simulink model "Half_car_model_susp_bump_tyre"  (R2025b)
settings: Solver=VariableStepAuto  StartTime=0.0  StopTime=25  RelTol=1e-3
values from neighbouring files (symbols this model uses):
  A_N = double(vpa(subs(A_0, symbol_vars , numeric_vals), 6))    [half_car_active_suspensions_bump.m]    (also in prova_ordinata.m = vpa(subs(A_0, vars , par), 6))
  B1_N = double(vpa(subs(B1_0, symbol_vars , numeric_vals), 6))    [half_car_active_suspensions_bump.m]    (also in prova_ordinata.m = vpa(subs(B1_0, vars , par), 6))
  B2_N = double(vpa(subs(B2_0, symbol_vars , numeric_vals), 6))    [half_car_active_suspensions_bump.m]    (also in prova_ordinata.m = vpa(subs(B2_0, vars , par), 6))
  C_N = double(vpa(subs(C_0, symbol_vars , numeric_vals), 6))    [half_car_active_suspensions_bump.m]    (also in prova_ordinata.m = vpa(subs(C_0, vars , par), 6))
  CE_N = double(vpa(subs(CE_0, symbol_vars , numeric_vals), 6))    [half_car_active_suspensions_bump.m]    (also in prova_ordinata.m = vpa(subs(CE_0, vars , par), 6))
  D1_N = double(vpa(subs(D1_0, symbol_vars , numeric_vals), 6))    [half_car_active_suspensions_bump.m]    (also in prova_ordinata.m = vpa(subs(D1_0, vars , par), 6))
  D2_N = double(vpa(subs(D2_0, symbol_vars , numeric_vals), 6))    [half_car_active_suspensions_bump.m]    (also in prova_ordinata.m = vpa(subs(D2_0, vars , par), 6))
  DE2_N = double(vpa(subs(DE2_0, symbol_vars , numeric_vals), 6))    [half_car_active_suspensions_bump.m]    (also in prova_ordinata.m = vpa(subs(DE2_0, vars , par), 6))
  Ko = lqr(A_reg', C_N', Q_kalman, R_kalman)'    [half_car_active_suspensions_bump.m]
  Ks = [Ks_c, zeros(2, 4)]    [half_car_active_suspensions_bump.m]
  Ks_obs = -[Ks_lqr_8, zeros(2, 4)]    [half_car_active_suspensions_bump.m]
  par_numeric = [m, kf, kr, betaf, betar, ell0, g, df, dr, J, mwf, mwr, ktf, ktr, hcg]    [half_car_active_suspensions_bump.m]
  rear_bump_time_delay = (df + dr) / vehicle_speed    (= 0.165)    [half_car_active_suspensions_bump.m]
  u0 = [0; 0]    [half_car_active_suspensions_bump.m]    (also in prova_ordinata.m = [0; k * Delta0 * (df - dr)])
  vehicle_speed = 20    [half_car_active_suspensions_bump.m]
  x0 = [  Delta0_num + Delta0_W_num ... (first row only)    [half_car_active_suspensions_bump.m]    (also in prova_ordinata.m = [Delta0)
  x0_lin = [ ... (first row only)    [half_car_active_suspensions_bump.m]
libraries: simulink x1
settings Model: LastModifiedBy=mario

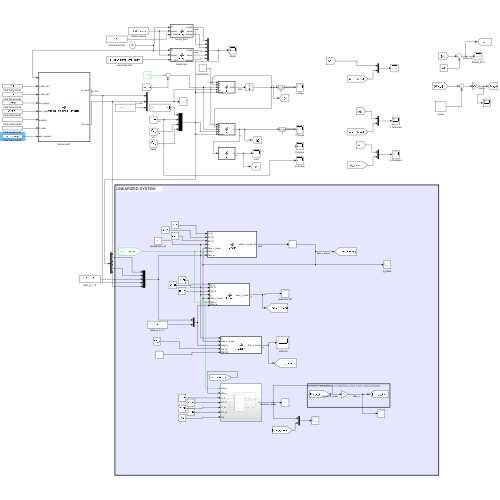
[thumbnail: Simulink's stored preview of the top-level diagram]
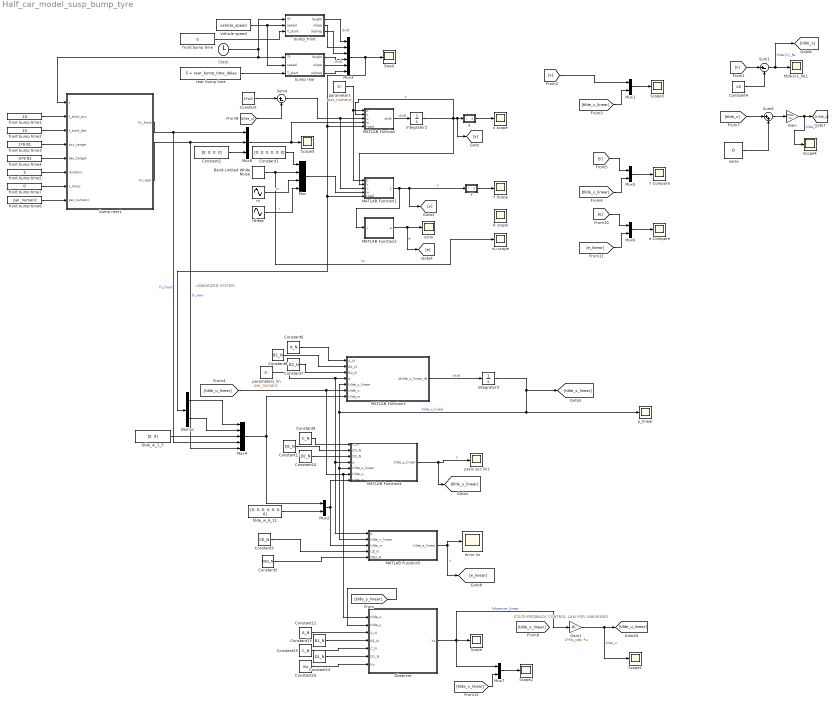
== system Half_car_model_susp_bump_tyre ==
  note: STATE-FEEDBACK CONTROL LAW FOR LINEARISED
  note: LINEARIZED SYSTEM
  " error lin" : Scope
      settings: ActiveDisplayYMinimum=-1  ActiveDisplayYMaximum=1  DataLoggingVariableName=ScopeData8
  Band-Limited White Noise : simulink/Sources/Band-Limited White Noise  Cov="1*[0.00001*1e-2; 0.00001*1e-2;  0.00001*1e-2; 0.00001*1e-2; 0.00001*1e-2]"  Ts=1e-2  seed=[23341; 31826; 11111; 81818; 00001]
  Clock : Clock
  Constant : Constant  Value=1*u0
  Constant1 : Constant  Value=[0; 0; 0; 0; 0; 0]
  Constant10 : Constant  Value=D2_N
  Constant11 : Constant  Value=D1_N
  Constant12 : Constant  Value=A_N
  Constant13 : Constant  Value=B1_N
  Constant14 : Constant  Value=D1_N
  Constant15 : Constant  Value=C_N
  Constant16 : Constant  Value=Ko
  Constant2 : Constant  Value=[0; 0; 0; 0]
  Constant3 : Constant  Value=CE_N
  Constant4 : Constant  Value=x0
  Constant5 : Constant  Value=DE2_N
  Constant6 : Constant  Value=A_N
  Constant7 : Constant  Value=B2_N
  Constant8 : Constant  Value=B1_N
  Constant9 : Constant  Value=C_N
  Demux : Demux  Outputs=6
  Gain : Gain  Gain=0*Ks  Multiplication=Matrix(K*u)
  Gain1 : Gain  Gain=1*Ks_obs  Multiplication=Matrix(K*u)
  Integrator2 : Integrator  InitialCondition=x0
  Integrator3 : Integrator  InitialCondition=x0_lin
  MATLAB Function : MATLAB Function  TreatAsAtomicUnit=on
  MATLAB Function1 : MATLAB Function  TreatAsAtomicUnit=on
  MATLAB Function2 : MATLAB Function  TreatAsAtomicUnit=on
  MATLAB Function3 : MATLAB Function  TreatAsAtomicUnit=on
  MATLAB Function4 : MATLAB Function  TreatAsAtomicUnit=on
  MATLAB Function5 : MATLAB Function  TreatAsAtomicUnit=on
  Mux : Mux
  Mux{1..2,5..7} (5 alike) : Mux  Inputs=2
  Mux3 : Mux  Inputs=6
  Mux4 : Mux  Inputs=5
  Mux8 : Mux  Inputs=3
  Observer : Subsystem
  R scope : Scope
      settings: ActiveDisplayYMinimum=-1  ActiveDisplayYMaximum=1  DataLoggingVariableName=ScopeData5
  Road : Scope
      settings: ActiveDisplayYMinimum=-0.39269908169872414  ActiveDisplayYMaximum=0.39269908169872414
  Scope{,1..5} (6 alike) : Scope
      Scope settings: ActiveDisplayYMinimum=-0.77419611103680575  ActiveDisplayYMaximum=0.44831124007175333  DataLoggingVariableName=ScopeData13
      Scope1 settings: ActiveDisplayYMinimum=-73646.15665947643  ActiveDisplayYMaximum=127134.62422776494  DataLoggingVariableName=ScopeData14
      Scope2 settings: ActiveDisplayYMinimum=-1  ActiveDisplayYMaximum=1  DataLoggingVariableName=ScopeData15
      Scope3 settings: ActiveDisplayYMinimum=-0.11890530130314077  ActiveDisplayYMaximum=0.069183222556784107
      Scope4 settings: ActiveDisplayYMinimum=-1  ActiveDisplayYMaximum=1  DataLoggingVariableName=ScopeData16
      Scope5 settings: ActiveDisplayYMinimum=-18087.1875  ActiveDisplayYMaximum=15634.6875  DataLoggingVariableName=ScopeData17
  Sum1 : Sum  Inputs=|+-
  Sum4 : Sum  Inputs=|+-
  Sum6 : Sum  Inputs=|++
  Vehicle speed : Constant  Value=vehicle_speed  VectorParams1D=off
  X : Subsystem
  Y : Subsystem
  Y Compare : Scope
      settings: ActiveDisplayYMinimum=-9.06978679583773  ActiveDisplayYMaximum=22.15478865739642  DataLoggingVariableName=ScopeData11
  Y Scope : Scope
      settings: ActiveDisplayYMinimum=-1  ActiveDisplayYMaximum=1  DataLoggingVariableName=ScopeData3
  bump rear : MATLAB Function  TreatAsAtomicUnit=on
  bump rear1 : MATLAB Function  TreatAsAtomicUnit=on
  bump_front : MATLAB Function  TreatAsAtomicUnit=on
  e Compare : Scope
      settings: ActiveDisplayYMinimum=-0.3208309292462625  ActiveDisplayYMaximum=0.34771769859425983  DataLoggingVariableName=ScopeData12
  "error " : Scope
      settings: ActiveDisplayYMinimum=-1  ActiveDisplayYMaximum=1  DataLoggingVariableName=ScopeData6
  front bump time : Constant  Value=5  VectorParams1D=off
  front bump time1 : Constant  Value=10  VectorParams1D=off
  front bump time2 : Constant  Value=15  VectorParams1D=off
  front bump time3 : Constant  Value=1*9.81  VectorParams1D=off
  front bump time4 : Constant  Value=-2*9.81  VectorParams1D=off
  front bump time5 : Constant  Value=3  VectorParams1D=off
  front bump time6 : Constant  Value=par_numeric  VectorParams1D=off
  front bump time7 : Constant  Value=0  VectorParams1D=off
  noise : Constant  Value=0
  nu scope : Scope
      settings: DataLoggingVariableName=ScopeData7
  p_linear : Scope
      settings: ActiveDisplayYMinimum=-0.03749851288711617  ActiveDisplayYMaximum=0.066646245320476569  DataLoggingVariableName=ScopeData9
  parameters : Constant  Value=par_numeric  VectorParams1D=off
  parameters_lin : Constant  Value=par_numeric
  rear bump time : Constant  Value=5 + rear_bump_time_delay  VectorParams1D=off
  rtheta : Sin  Amplitude=0  Frequency=0  SampleTime=0
  rz : Sin  Amplitude=0  Frequency=0  SampleTime=0
  tilde_w_1_5 : Constant  Value=[0; 0]
  tilde_w_6_11 : Constant  Value=[0; 0; 0; 0; 0; 0; 0]
  "tilde{x}_NL1" : Scope
      settings: ActiveDisplayYMinimum=-4.93552  ActiveDisplayYMaximum=2.55492  DataLoggingVariableName=ScopeData4
  x scope : Scope
      settings: ActiveDisplayYMinimum=-0.070953530518173463  ActiveDisplayYMaximum=0.13842945478834703  DataLoggingVariableName=ScopeData2
  yaxis acc lin1 : Scope
      settings: ActiveDisplayYMinimum=-1  ActiveDisplayYMaximum=1  DataLoggingVariableName=ScopeData10
  wires:
  Mux3/1 -> MATLAB Function/5(road), Demux/1, MATLAB Function1/5(road), Road/1
  bump_front/1(height) -> Mux3/1  "dxdt"
  Constant/1 -> Sum4/1
  Sum4/1 -> MATLAB Function1/3(u), MATLAB Function/3(u)
  MATLAB Function/1(dxdt) -> Integrator2/1  "dxdt"
  MATLAB Function1/1(y) -> Y/1(i), [y], MATLAB Function2/1(y)  "y"
  rtheta/1 -> Mux/4  "r"
  parameters/1 -> MATLAB Function1/1(p), MATLAB Function/1(p)
  Band-Limited White Noise/1 -> nu scope/1, Mux/2  "nu"
  rz/1 -> Mux/3  "rz"
  Mux/1 -> MATLAB Function1/4(w)
  MATLAB Function2/1(e) -> [e], "error "/1  "e"
  Sum6/1 -> Gain/1
  [tilde_x] -> Sum6/1
  [x] -> Sum1/1
  Constant4/1 -> Sum1/2
  Sum1/1 -> [tilde_x], "tilde{x}_NL1"/1  "tilde{x}_NL"
  noise/1 -> Sum6/2
  [tilde_x_linear] -> Mux1/2
  Gain/1 -> Scope4/1, [tilde_u]  "tilde_u"
  Mux1/1 -> Scope3/1
  [tilde_u] -> Sum4/2
  Integrator2/1 -> [x], X/1(i), MATLAB Function1/2(x), MATLAB Function/2(x)  "x"
  X/1(o) -> x scope/1
  Y/1(o) -> Y Scope/1
  tilde_w_6_11/1 -> Mux2/2
  parameters_lin/1 -> MATLAB Function3/4(p), MATLAB Function5/1(p), MATLAB Function4/4(p)
  [tilde_u_linear] -> MATLAB Function3/6(tilde_u), Observer/1(tilde_u), MATLAB Function4/6(tilde_u)
  Gain1/1 -> Scope1/1, [tilde_u_linear]  "tilde_u"
  MATLAB Function4/1(tilde_y_linear) -> [tilde_y_linear], yaxis acc lin1/1  "y"
  Mux2/1 -> MATLAB Function4/7(tilde_w), MATLAB Function5/3(tilde_w)
  MATLAB Function5/1(tilde_e_linear) -> " error lin"/1, [e_linear]  "y"
  Constant3/1 -> MATLAB Function5/4(CE_N)
  Constant5/1 -> MATLAB Function5/5(DE2_N)
  Constant7/1 -> MATLAB Function3/3(B2_N)
  Constant6/1 -> MATLAB Function3/1(A_N)
  Constant8/1 -> MATLAB Function3/2(B1_N)
  Constant10/1 -> MATLAB Function4/3(D2_N)
  Constant11/1 -> MATLAB Function4/2(D1_N)
  Constant9/1 -> MATLAB Function4/1(C_N)
  Mux4/1 -> MATLAB Function3/7(tilde_w), Mux2/1
  tilde_w_1_5/1 -> Mux4/3
  Demux/2 -> Mux4/1
  Demux/5 -> Mux4/2
  MATLAB Function3/1(dtilde_x_linear_dt) -> Integrator3/1  "dxdt"
  Integrator3/1 -> p_linear/1, MATLAB Function3/5(tilde_x_linear), MATLAB Function5/2(tilde_x_linear), MATLAB Function4/5(tilde_x_linear), [tilde_x_linear]  "tilde_x_linear"
  [y] -> Mux5/1
  Mux5/1 -> Y Compare/1
  [tilde_y_linear] -> Mux5/2
  Mux6/1 -> e Compare/1
  [e] -> Mux6/1
  [e_linear] -> Mux6/2
  [tilde_y_linear] -> Observer/2(tilde_y)
  Observer/1(Yo) -> Mux7/1, Gain1/1, Scope/1  "Yobserver_linear"
  Constant16/1 -> Observer/7(Ko)
  Constant14/1 -> Observer/6(D1_N)
  Constant15/1 -> Observer/5(C_N)
  Constant13/1 -> Observer/4(B1_N)
  Constant12/1 -> Observer/3(A_N)
  Mux7/1 -> Scope2/1
  [x] -> Mux1/1
  bump_front/2(slope) -> Mux3/2
  bump_front/3(alphag) -> Mux3/3
  bump rear/1(height) -> Mux3/4  "dxdt"
  bump rear/2(slope) -> Mux3/5
  bump rear/3(alphag) -> Mux3/6
  Vehicle speed/1 -> bump rear/2(speed), bump_front/2(speed)
  Clock/1 -> bump_front/1(Tf), bump rear/1(Tf), bump rear1/1(t)
  front bump time/1 -> bump_front/3(T_start)
  rear bump time/1 -> bump rear/3(T_start)
  [tilde_x_linear] -> Mux7/2
  front bump time1/1 -> bump rear1/2(t_start_acc)
  front bump time2/1 -> bump rear1/3(t_start_dec)
  front bump time3/1 -> bump rear1/4(acc_target)
  front bump time4/1 -> bump rear1/5(dec_target)
  front bump time5/1 -> bump rear1/6(duration)
  front bump time6/1 -> bump rear1/8(par_numeric)
  bump rear1/1(Fx_front) -> Mux4/4, Mux8/1  "fx_front"
  bump rear1/2(Fx_rear) -> Mux4/5, Mux8/2  "fx_rear"
  Constant1/1 -> Mux/1
  Constant2/1 -> Mux8/3
  Mux8/1 -> Scope5/1, MATLAB Function/4(w)
  front bump time7/1 -> bump rear1/7(t_ramp)

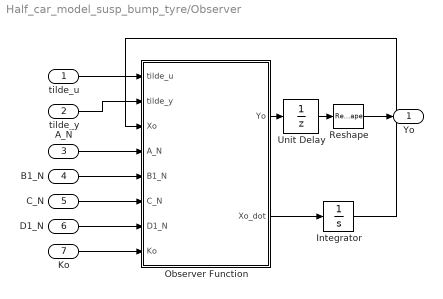
== system Half_car_model_susp_bump_tyre/Observer ==
  tilde_u : Inport
  tilde_y : Inport  Port=2
  A_N : Inport  Port=3
  B1_N : Inport  Port=4
  C_N : Inport  Port=5
  D1_N : Inport  Port=6
  Ko : Inport  Port=7
  Integrator : Integrator  InitialCondition=x0_lin
  Observer Function : MATLAB Function  TreatAsAtomicUnit=on
  Reshape : Reshape  OutputDimensionality=Customize  OutputDimensions=[12]
  Unit Delay : UnitDelay  SampleTime=0.01  HasFrameUpgradeWarning=on
  Yo : Outport
  wires:
  Observer Function/2(Xo_dot) -> Integrator/1
  Integrator/1 -> Observer Function/3(Xo)
  tilde_u/1 -> Observer Function/1(tilde_u)
  tilde_y/1 -> Observer Function/2(tilde_y)
  A_N/1 -> Observer Function/4(A_N)
  B1_N/1 -> Observer Function/5(B1_N)
  C_N/1 -> Observer Function/6(C_N)
  D1_N/1 -> Observer Function/7(D1_N)
  Ko/1 -> Observer Function/8(Ko)
  Reshape/1 -> Yo/1
  Observer Function/1(Yo) -> Unit Delay/1
  Unit Delay/1 -> Reshape/1

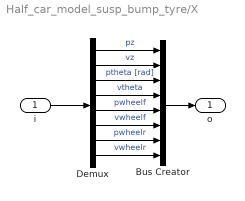
== system Half_car_model_susp_bump_tyre/X ==
  i : Inport
  Bus Creator : BusCreator  Inputs=8
  Demux : Demux  Outputs=8
  o : Outport
  wires:
  Demux/8 -> Bus Creator/8  "vwheelr"
  Demux/4 -> Bus Creator/4  "vtheta"
  Demux/1 -> Bus Creator/1  "pz"
  Demux/2 -> Bus Creator/2  "vz"
  Demux/5 -> Bus Creator/5  "pwheelf"
  Demux/3 -> Bus Creator/3  "ptheta [rad]"
  Demux/7 -> Bus Creator/7  "pwheelr"
  Demux/6 -> Bus Creator/6  "vwheelf"
  i/1 -> Demux/1
  Bus Creator/1 -> o/1

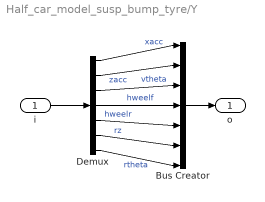
== system Half_car_model_susp_bump_tyre/Y ==
  i : Inport
  Bus Creator : BusCreator  Inputs=7
  Demux : Demux  Outputs=7
  o : Outport
  wires:
  Demux/4 -> Bus Creator/4  "hweelf"
  Demux/1 -> Bus Creator/1  "xacc"
  Demux/2 -> Bus Creator/2  "zacc"
  Demux/3 -> Bus Creator/3  "vtheta"
  i/1 -> Demux/1
  Bus Creator/1 -> o/1
  Demux/7 -> Bus Creator/7  "rtheta"
  Demux/6 -> Bus Creator/6  "rz"
  Demux/5 -> Bus Creator/5  "hweelr"

== matlab function Half_car_model_susp_bump_tyre/Observer/Observer Function ==
  data: tilde_u input; tilde_y input; Yo output; Xo_dot output; Xo input; A_N input; B1_N input; C_N input; D1_N input; Ko input
function [Yo, Xo_dot] = fcn(tilde_u, tilde_y, Xo, A_N, B1_N, C_N, D1_N, Ko)
    % tilde_u: Ingressi di controllo [2x1] (u1, u2)
    % tilde_y: Misure dai sensori [5x1] (ax, az, vtheta, s1, s3)
    % Xo:      Stato stimato attuale [12x1]
    % Ko:      Guadagno dell'osservatore [12x5]
    
    %% 1. Calcolo dell'uscita stimata (Cosa l'osservatore "pensa" di leggere)
    % y_hat = C * x_stimato + D * u
    tilde_y_hat = C_N * Xo + D1_N * tilde_u;
    
    %% 2. Calcolo dell'errore di stima (Residuo)
    % Differenza tra misura reale del sensore e misura prevista dal modello
    e_y = tilde_y - tilde_y_hat;
    
    %% 3. Dinamica dell'Observer (Equazione di Luenberger)
    % Xo_dot = A*Xo + B*u + Ko*(y - y_hat)
    % Il termine Ko * e_y è quello che corregge lo stato verso la realtà
    Xo_dot = A_N * Xo + B1_N * tilde_u + Ko * e_y;
    
    %% 4. Uscita dell'Observer
    % In questo caso Yo è lo stato stimato completo che va allo stabilizzatore
    % Non serve reshape se Xo è già un vettore colonna 12x1
    Yo = Xo; 
    
end

== matlab function Half_car_model_susp_bump_tyre/bump rear1 ==
  data: Fx_front output; Fx_rear output; t input; t_start_acc input; t_start_dec input; acc_target input; dec_target input; duration input; t_ramp input; par_numeric input
function [Fx_front, Fx_rear] = vehicle_dynamics_corrected(t, t_start_acc, t_start_dec, acc_target, dec_target, duration, t_ramp, par_numeric)
    % Estrazione
    m_total = par_numeric(1); % 2500 kg
    
    % Dividiamo la massa per 2: il modello Half-Car rappresenta un solo lato
    m_half = m_total / 2; 

    ax = 0;
    % ... (Logica della rampa identica a prima) ...
    if t >= t_start_acc && t < (t_start_acc + duration)
        rel_t = t - t_start_acc;
        if rel_t < t_ramp, ax = acc_target * (rel_t / t_ramp);
        elseif rel_t > (duration - t_ramp), ax = acc_target * ((duration - rel_t) / t_ramp);
        else, ax = acc_target; end
    elseif t >= t_start_dec && t < (t_start_dec + duration)
        rel_t = t - t_start_dec;
        if rel_t < t_ramp, ax = dec_target * (rel_t / t_ramp);
        elseif rel_t > (duration - t_ramp), ax = dec_target * ((duration - rel_t) / t_ramp);
        else, ax = dec_target; end
    end

    % Forza per LATO (Half-Car)
    Fx_side = m_half * ax;

    % Ripartizione
    if ax > 0
        Fx_front = 0;
        Fx_rear = Fx_side; % Ora sarà ~12.25 kN a 1g
    else
        Fx_front = Fx_side * 0.6; 
        Fx_rear = Fx_side * 0.4;
    end
end

== matlab function Half_car_model_susp_bump_tyre/MATLAB Function1 ==
  data: p input; x input; u input; y output; w input; road input
function y = h(p,x, u, w, road)

%% parameters
m = p(1);      % [kg] mass
k = p(2);    % [N/m] spring stiffness
beta = p(3);   % [N/(m/s)] damper coeff.
ell0 = p(4);   % [m] 0-load lenght
g = p(5);   % [m/s^2] gravity acceleration
df = p(6);     % [m] distance between center of mass and front
dr = p(7);     % [m] distance between center of mass and rear
J = p(8);      % [kg*m^2] Moment of interti
mwf = p(9);     %[kg] massa ruote AV (asse completo)
mwr = p(10);    %[kg] massa ruote AP (asse completo)
ktf = p(11);   %[N/m] rigidezza pneumatici AV (asse)
ktr = p(12);  %[N/m] rigidezza pneumatici AP (asse)

%% state
pz = x(1);        % [m] heigth of the center of mass of the car 
vz = x(2);        % [m/s] speed of the center of mass of the car 
ptheta = x(3);    % [Rad] pitch angle of the car 
vtheta = x(4);    % [Rad/s] angular speed of the car 
hwheelf = x(5);
dhwheelf = x(6);
hwheelr = x(7);
dhwheelr = x(8);


zroad_f = road(1);
thetaroad_f = road(2);
alphag_f = road(3);

zroad_r = road(4);    
thetaroad_r = road(5); 
alphag_r = w(6);

%% disturbance
zroad_f_dot = w(1);
zroad_r_dot = w(2);
% alphag_f = w(3);
% alphag_r = w(4);
fwfront = w(5);
fwrear = w(6);

%todo: Vedere se servono due disturbi 

%% state evolution
 
s1 = (pz-hwheelf)+df*(sin(ptheta)-sin(thetaroad_f)); % height of front suspension
s3 = (pz-hwheelr)-dr*(sin(ptheta)-sin(thetaroad_r)); % height of rear suspension

% s2 = (vz-dhwheelf)+df*(vtheta*cos(ptheta)-thetaroad_f*cos(thetaroad_f)); % height speed of front suspension
% s4 = (vz-dhwheelr)-dr*(vtheta*cos(ptheta)-thetaroad_r*cos(thetaroad_r)); % height speed of rear suspension

s2 = (vz-dhwheelf)+df*(vtheta*cos(ptheta)-alphag_f*cos(thetaroad_f)); % height speed of front suspension
s4 = (vz-dhwheelr)-dr*(vtheta*cos(ptheta)-alphag_r*cos(thetaroad_r)); % height speed of rear suspension

lf = s1 + ell0;
lr = s3 + ell0;

%% Forze sospensioni & pneumatici
fsf = -k*s1 - beta*s2;      % sospensione anteriore
fsr = -k*s3 - beta*s4;      % sospensione posteriore

ftf =  ktf*(zroad_f - hwheelf); % pneumatico anteriore (no damping)
ftr =  ktr*(zroad_r - hwheelr); % pneumatico posteriore (no damping)

fmgf = - mwf * g;
fmgr = - mwf * g;

%% Ripartizione attuatori u1,u2 -> forze su body alle estremità
% [faf + far = u1;   df*faf - dr*far = u2]
faf = (u(2) + dr*u(1))/(df + dr);      % forza attuatore anteriore
far = (df*u(1) - u(2))/(df + dr);      % forza attuatore posteriore

%% Dinamica: corpo
f2 = -g + (fsf + fsr + u(1))/m;                                     % acc. verticale
f4 = (df*fsf - dr*fsr + u(2) + fwfront*lf + fwrear*lr)/J;           % pitch

%% Dinamica: ruote (masse non sospese)
% segno: su ruota, verso +z è (forza pneumatico - forza sospensione - attuatore locale)
f_wf = (ftf - fsf - faf + fmgf)/mwf;   % acc. ruota ant
f_wr = (ftr - fsr - far + fmgr)/mwr;   % acc. ruota post


nuy = w(7);
nuz = w(7);
nug = w(7);
nuf = w(7);
nur = w(7);

%% reference
rz = w(8);
rtheta=w(9);


%% output
y = [sin(x(3))*(f2 + g) + cos(x(3)) * ((fwrear + fwfront) / m)+nuy; % h_xacc
     cos(x(3))*(f2 + g) - sin(x(3)) * ((fwrear + fwfront) / m)+nuz; % h_zacc  se facciamo cosi ci da in condizioni stazionarie Zaxisacc=9.81, se vogliamo il valore negativo mettere "-" davanti a coseno 
     x(4)+nug;                                                      % h_vtheta
     s1+nuf;                                                        % h_hweelf
     s3+nur;                                                        % h_hweelf
     rz;                                                            % h_rz
     rtheta];                                                       % h_rtheta
end

== matlab function Half_car_model_susp_bump_tyre/MATLAB Function ==
  data: p input; x input; u input; dxdt output; w input; road input
function dxdt = f(p,x,u,w,road)
%% parameters (Aggiornati per 15 parametri)
m      = p(1);    
kf     = p(2);    % Rigidezza anteriore
kr     = p(3);    % Rigidezza posteriore
betaf  = p(4);    % Smorzamento anteriore
betar  = p(5);    % Smorzamento posteriore
ell0   = p(6);    
g      = p(7);    
df     = p(8);    
dr     = p(9);    
J      = p(10);    
mwf    = p(11);    
mwr    = p(12);   
ktf    = p(13);   
ktr    = p(14);
hcg    = p(15);   % Altezza del baricentro

%% state
pz      = x(1); vz      = x(2);
ptheta  = x(3); vtheta  = x(4);
hwheelf = x(5); dhwheelf = x(6);
hwheelr = x(7); dhwheelr = x(8);

% Road input
zroad_f = road(1);
zroad_r = road(4);

%% disturbance / Longitudinal Forces
% Usiamo w(1) e w(2) come forze longitudinali (Fx) per coerenza con l'assegnazione precedente
Fxf = w(1); 
Fxr = w(2); 
F_tot_x = Fxf + Fxr; 

%% Equazioni cinematiche
s1 = (pz + df * sin(ptheta)) - hwheelf; 
s3 = (pz - dr * sin(ptheta)) - hwheelr;
s2 = vz + df * vtheta * cos(ptheta) - dhwheelf;
s4 = vz - dr * vtheta * cos(ptheta) - dhwheelr;

%% Forze sospensioni & pneumatici (Modificate con kf, kr, betaf, betar)
fsf = -kf*s1 - betaf*s2;      
fsr = -kr*s3 - betar*s4;      

ftf =  ktf*(zroad_f - hwheelf); 
ftr =  ktr*(zroad_r - hwheelr); 
fmgf = - mwf * g;
fmgr = - mwr * g; 

%% Ripartizione attuatori (Input attivi u1, u2)
faf = (u(2) + dr*u(1))/(df + dr);      
far = (df*u(1) - u(2))/(df + dr);      

%% Dinamica: corpo
% Accelerazione verticale
f2 = -g + (fsf + fsr + faf + far)/m;                  

% Dinamica Pitch (f4): Momento totale inclusa la spinta longitudinale hcg
f4 = (df*(fsf + faf) - dr*(fsr + far) + F_tot_x * hcg) / J;             

%% Dinamica: ruote
f_wf = (ftf - fsf - faf + fmgf)/mwf;   
f_wr = (ftr - fsr - far + fmgr)/mwr;   
        
dxdt = [ ...
    vz;                   
    f2;                   
    vtheta;               
    f4;                   
    dhwheelf;             
    f_wf;                 
    dhwheelr;             
    f_wr ];               
end

== matlab function Half_car_model_susp_bump_tyre/MATLAB Function2 ==
  data: y input; e output
function e = E(y)

df = 1;     % [m] distance between center of mass and front
dr = 1;     % [m] distance between center of mass and rear


yy = y(1); % output of h block yaxisacc 
yz = y(2); % output of h block zaxisacc 
yg = y(3); % output of h block gyro
yf = y(4); % output of h block pot. front
yr = y(5); % output of h block pot. rear
 
%% ref
rz = y(6);
rtheta = y(7);

e = [
    (yf*dr+yr*df)/(dr+df)-rz; 
    asin((yy)/(sqrt(yy^2+yz^2)))-rtheta];
end

== matlab function Half_car_model_susp_bump_tyre/MATLAB Function3 ==
  data: A_N input; B1_N input; B2_N input; p input; tilde_x_linear input; tilde_u input; dtilde_x_linear_dt output; tilde_w input
function dtilde_x_linear_dt = Linear(A_N, B1_N, B2_N, p,tilde_x_linear,tilde_u,tilde_w)

dtilde_x_linear_dt = A_N*tilde_x_linear+B1_N*tilde_u+B2_N*tilde_w;
end

== matlab function Half_car_model_susp_bump_tyre/MATLAB Function4 ==
  data: C_N input; D1_N input; D2_N input; p input; tilde_x_linear input; tilde_u input; tilde_y_linear output; tilde_w input
function tilde_y_linear = Linear(C_N, D1_N, D2_N, p,tilde_x_linear,tilde_u,tilde_w)

% 
% %% parameters
% m = p(1);      % [kg] mass
% k = p(2);    % [N/m] spring stiffness
% beta = p(3);   % [N/(m/s)] damper coeff.
% ell0 = p(4);   % [m] 0-load lenght
% g = p(5);   % [m/s^2] gravity acceleration
% df = p(6);     % [m] distance between center of mass and front
% dr = p(7);     % [m] distance between center of mass and rear
% J = p(8);      % [kg*m^2] Moment of interti
% 
% 
% 
% C = [0, 0, g, 0, 0, 0;
%     -2*k/m, -2*beta/m, -k*(df-dr)/m, -beta*(df-dr)/m, k*(df-dr)/m, beta*(df-dr)/m;
%     0, 0, 0, 1, 0, 0;
%     1, 0, df, 0, -df, 0;
%     1, 0, -dr, 0, dr, 0];
% 
% 
% D1 = [0,0;
%      1/m, 0;
%      0,0;
%      0,0;
%      0,0];
% 
% D2 = [0,0,1/m,1/m,1,0,0,0,0,0,0;
%       0,0,0,0,0,1,0,0,0,0,0;
%       0,0,0,0,0,0,1,0,0,0,0;
%       0,0,0,0,0,0,0,1,0,0,0;
%       0,0,0,0,0,0,0,0,1,0,0];

%% state evolution
% tilde_y_linear = C*tilde_x_linear+D1*tilde_u+D2*tilde_w;

tilde_y_linear = C_N*tilde_x_linear+D1_N*tilde_u+D2_N*tilde_w;
end

== matlab function Half_car_model_susp_bump_tyre/MATLAB Function5 ==
  data: p input; tilde_x_linear input; tilde_e_linear output; tilde_w input; CE_N input; DE2_N input
function tilde_e_linear = Linear(p,tilde_x_linear,tilde_w, CE_N, DE2_N)

% 
% %% parameters
% m = p(1);      % [kg] mass
% k = p(2);    % [N/m] spring stiffness
% beta = p(3);   % [N/(m/s)] damper coeff.
% ell0 = p(4);   % [m] 0-load lenght
% g = p(5);   % [m/s^2] gravity acceleration
% df = p(6);     % [m] distance between center of mass and front
% dr = p(7);     % [m] distance between center of mass and rear
% J = p(8);      % [kg*m^2] Moment of interti
% 
% 
% 
% Ce = [1,0,0,0,0,0;
%       0,0,1,0,0,0];
% 
% 
% 
% De2 = [0,0,0,0,0,0,0,dr/(dr+df),df/(dr+df),-1,0;
%        0,0, 1/(m*g),1/(m*g),1/g,0,0,0,0,0,-1];


%% state evolution
% tilde_e_linear = Ce*tilde_x_linear+De2*tilde_w;

tilde_e_linear = CE_N*tilde_x_linear+DE2_N*tilde_w;
end

== matlab function Half_car_model_susp_bump_tyre/bump rear ==
  data: height output; slope output; Tf input; alphag output; speed input; T_start input
function [height, slope, alphag] = bump(Tf, speed, T_start)
    % --- Parametri FISICI (fissi) ---
    a = 0.1;           % Ampiezza del bump (metri)
    lambda = 1;       % Lunghezza FISICA del bump (metri)
    V = speed;         % Velocità (m/s)
    
    % --- Definizione Intervallo Temporale ---
    % Il bump inizia a T_start e finisce quando il veicolo ha percorso lambda
    T1 = T_start;
    T2 = T1 + lambda/V;

    % Controllo se la ruota è sul dosso al tempo attuale Tf
    is_on_bump = (Tf >= T1) & (Tf <= T2);
    
    % --- Calcolo delle uscite ---
    % L'argomento del coseno deve dipendere dal tempo trascorso dall'inizio del bump
    % delta_t va da 0 a lambda/V
    delta_t = Tf - T1;
    
    % Frequenza angolare basata sulla velocità e lunghezza d'onda
    omega = (2 * pi * V) / lambda;
    phi = omega * delta_t;
    
    % Altezza (m)
    height = (a/2) * (1 - cos(phi)) .* is_on_bump; 
    
    % Pendenza (dh/dt - velocità verticale in m/s)
    slope = (a/2) * omega .* sin(phi) .* is_on_bump; 
    
    % Accelerazione del profilo (d2h/dt2 - m/s^2)
    alphag = (a/2) * (omega^2) .* cos(phi) .* is_on_bump; 
end

== matlab function Half_car_model_susp_bump_tyre/bump_front ==
  data: height output; slope output; Tf input; alphag output; speed input; T_start input
function [height, slope, alphag] = bump(Tf, speed, T_start)
    % --- Parametri FISICI (fissi) ---
    a = 0.1;           % Ampiezza del bump (metri)
    lambda = 1;       % Lunghezza FISICA del bump (metri)
    V = speed;         % Velocità (m/s)
    
    % --- Definizione Intervallo Temporale ---
    % Il bump inizia a T_start e finisce quando il veicolo ha percorso lambda
    T1 = T_start;
    T2 = T1 + lambda/V;

    % Controllo se la ruota è sul dosso al tempo attuale Tf
    is_on_bump = (Tf >= T1) & (Tf <= T2);
    
    % --- Calcolo delle uscite ---
    % L'argomento del coseno deve dipendere dal tempo trascorso dall'inizio del bump
    % delta_t va da 0 a lambda/V
    delta_t = Tf - T1;
    
    % Frequenza angolare basata sulla velocità e lunghezza d'onda
    omega = (2 * pi * V) / lambda;
    phi = omega * delta_t;
    
    % Altezza (m)
    height = (a/2) * (1 - cos(phi)) .* is_on_bump; 
    
    % Pendenza (dh/dt - velocità verticale in m/s)
    slope = (a/2) * omega .* sin(phi) .* is_on_bump; 
    
    % Accelerazione del profilo (d2h/dt2 - m/s^2)
    alphag = (a/2) * (omega^2) .* cos(phi) .* is_on_bump; 
end
